simulink model "P4_F_sim"  (R2019a)
settings: Solver=VariableStepAuto  StartTime=0.0  StopTime=10.0  RelTol=1e-3
values from neighbouring files (symbols this model uses):
  A_AA = [ybb  yp+w0/u0 yr-1 g*ctt0/u0 ... (first row only)    [P3_F.m]
  B = [0    ydr ... (first row only)    [P3_F.m]
  bb_ref = 0.8    [P3_F.m]
  bb_stept = 10    [P3_F.m]
  C = eye(4)    [P3_F.m]
  D = zeros(4,2)    [P3_F.m]
  da0 = 0.58    [P3_F.m]
  damax = [-18 18]    [P3_F.m]
  deg = pi/180    (= 0.0174532925199)    [P3_F.m]
  dr0 = -0.01    [P3_F.m]
  drmax = [-23 23]    [P3_F.m]
  F = (CC*dcgain)^(-1)    [P3_F.m]
  K_lqr = lqr(A_AA,B,Q,R)    [P3_F.m]
  phi_ref = 15    [P3_F.m]
  phi_stept = 50    [P3_F.m]
libraries: simulink x4
settings Model: Creator=User  LastModifiedBy=User
settings DebuggingCC: SFMachineParentedDataDiag=error

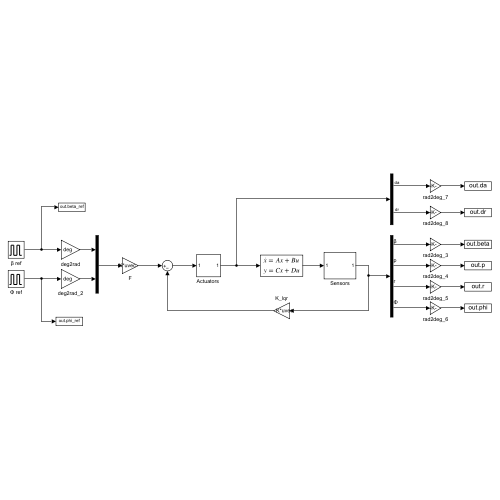
[thumbnail: Simulink's stored preview of the top-level diagram]
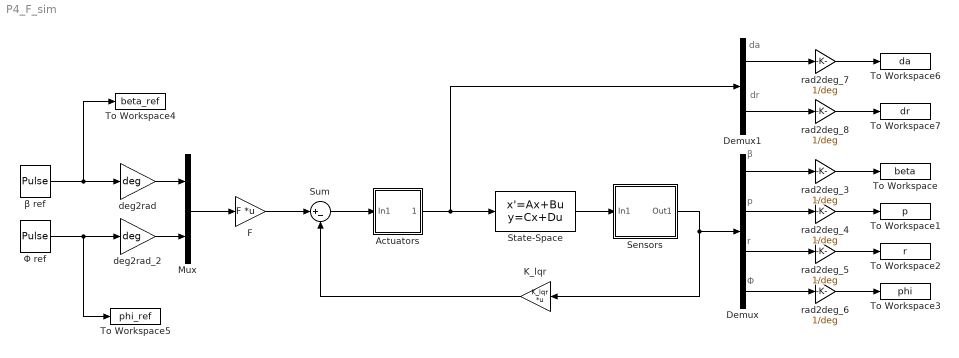
== system P4_F_sim ==
  note: r
  note: da
  note: p
  note: dr
  note: β
  note: Φ
  "Actuators " : Subsystem
  Demux : Demux
  Demux1 : Demux  Outputs=2
  F : Gain  Gain=F  Multiplication=Matrix(K*u) (u vector)
  K_lqr : Gain  Gain=K_lqr  Multiplication=Matrix(K*u) (u vector)
  Mux : Mux  Inputs=2
  Sensors : Subsystem
  State-Space : StateSpace  A=A_AA  B=B  C=C  D=D  InitialCondition=0
  Sum : Sum  Inputs=|+-
  To Workspace : ToWorkspace  VariableName=beta  SaveFormat=Timeseries  SampleTime=-1
  To Workspace1 : ToWorkspace  VariableName=p  SaveFormat=Timeseries  SampleTime=-1
  To Workspace2 : ToWorkspace  VariableName=r  SaveFormat=Timeseries  SampleTime=-1
  To Workspace3 : ToWorkspace  VariableName=phi  SaveFormat=Timeseries  SampleTime=-1
  To Workspace4 : ToWorkspace  VariableName=beta_ref  SaveFormat=Timeseries  SampleTime=-1
  To Workspace5 : ToWorkspace  VariableName=phi_ref  SaveFormat=Timeseries  SampleTime=-1
  To Workspace6 : ToWorkspace  VariableName=da  SaveFormat=Timeseries  SampleTime=-1
  To Workspace7 : ToWorkspace  VariableName=dr  SaveFormat=Timeseries  SampleTime=-1
  deg2rad : Gain  Gain=deg
  deg2rad_2 : Gain  Gain=deg
  rad2deg_{3..8} (6 alike) : Gain  Gain=1/deg
  Φ ref : DiscretePulseGenerator  PulseType=Time based  Amplitude=phi_ref  Period=100  PulseWidth=20  PhaseDelay=phi_stept
  β ref : DiscretePulseGenerator  PulseType=Time based  Amplitude=bb_ref  Period=100  PulseWidth=20  PhaseDelay=bb_stept
  wires:
  F/1 -> Sum/1
  Demux/2 -> rad2deg_4/1
  Demux/4 -> rad2deg_6/1
  Demux/3 -> rad2deg_5/1
  rad2deg_4/1 -> To Workspace1/1
  rad2deg_6/1 -> To Workspace3/1
  Demux1/1 -> rad2deg_7/1
  deg2rad/1 -> Mux/1
  rad2deg_7/1 -> To Workspace6/1
  K_lqr/1 -> Sum/2
  Mux/1 -> F/1
  Demux/1 -> rad2deg_3/1
  β ref/1 -> To Workspace4/1, deg2rad/1
  deg2rad_2/1 -> Mux/2
  rad2deg_8/1 -> To Workspace7/1
  Demux1/2 -> rad2deg_8/1
  rad2deg_5/1 -> To Workspace2/1
  rad2deg_3/1 -> To Workspace/1
  Φ ref/1 -> deg2rad_2/1, To Workspace5/1
  Sum/1 -> "Actuators "/1(In1)
  "Actuators "/1(Out1) -> Demux1/1, State-Space/1
  State-Space/1 -> Sensors/1(In1)
  Sensors/1(Out1) -> Demux/1, K_lqr/1

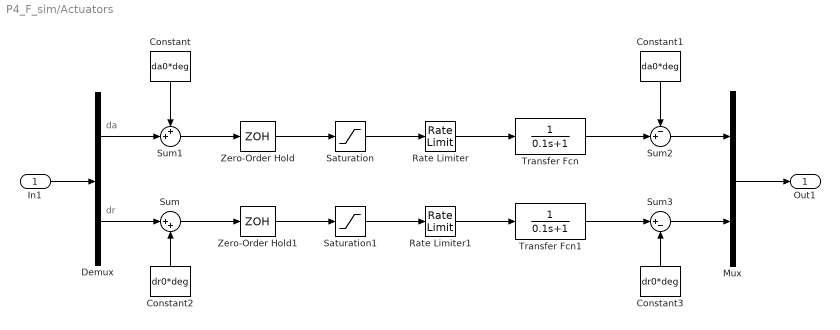
== system P4_F_sim/Actuators  ==
  note: da
  note: dr
  In1 : Inport
  Constant : Constant  Value=da0*deg
  Constant1 : Constant  Value=da0*deg
  Constant2 : Constant  Value=dr0*deg
  Constant3 : Constant  Value=dr0*deg
  Demux : Demux  Outputs=2
  Mux : Mux  Inputs=2
  Rate Limiter : RateLimiter  RisingSlewLimit=60*deg  FallingSlewLimit=-60*deg  SampleTimeMode=inherited
  Rate Limiter1 : RateLimiter  RisingSlewLimit=60*deg  FallingSlewLimit=-60*deg  SampleTimeMode=inherited
  Saturation : Saturate  UpperLimit=damax(2) * deg  LowerLimit=damax(1) * deg
  Saturation1 : Saturate  UpperLimit=drmax(2) * deg  LowerLimit=drmax(1) * deg
  Sum : Sum  Inputs=|++
  Sum1 : Sum  Inputs=++|
  Sum2 : Sum  Inputs=-+|
  Sum3 : Sum  Inputs=|+-
  Transfer Fcn : TransferFcn  Denominator=[0.1 1]
  Transfer Fcn1 : TransferFcn  Denominator=[0.1 1]
  Zero-Order Hold : ZeroOrderHold  SampleTime=0.025
  Zero-Order Hold1 : ZeroOrderHold  SampleTime=0.025
  Out1 : Outport
  wires:
  In1/1 -> Demux/1
  Zero-Order Hold/1 -> Saturation/1
  Zero-Order Hold1/1 -> Saturation1/1
  Saturation/1 -> Rate Limiter/1
  Saturation1/1 -> Rate Limiter1/1
  Rate Limiter/1 -> Transfer Fcn/1
  Rate Limiter1/1 -> Transfer Fcn1/1
  Mux/1 -> Out1/1
  Sum/1 -> Zero-Order Hold1/1
  Demux/2 -> Sum/1
  Sum1/1 -> Zero-Order Hold/1
  Demux/1 -> Sum1/2
  Transfer Fcn/1 -> Sum2/2
  Sum2/1 -> Mux/1
  Transfer Fcn1/1 -> Sum3/1
  Sum3/1 -> Mux/2
  Constant/1 -> Sum1/1
  Constant1/1 -> Sum2/1
  Constant3/1 -> Sum3/2
  Constant2/1 -> Sum/2

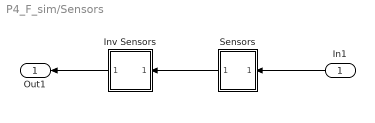
== system P4_F_sim/Sensors ==
  In1 : Inport
  Inv Sensors : Subsystem
  Sensors : Subsystem
  Out1 : Outport
  wires:
  Sensors/1(Out1) -> Inv Sensors/1(Input)
  Inv Sensors/1(Out1) -> Out1/1
  In1/1 -> Sensors/1(In1)

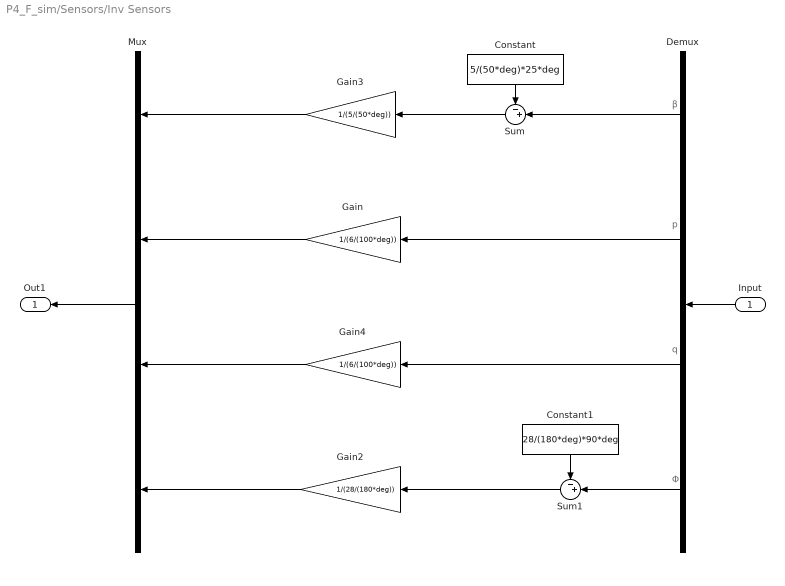
== system P4_F_sim/Sensors/Inv Sensors ==
  note: p
  note: β
  note: Φ
  note: q
  Input : Inport
  Constant : Constant  Value=5/(50*deg)*25*deg
  Constant1 : Constant  Value=28/(180*deg)*90*deg
  Demux : Demux
  Gain : Gain  Gain=1/(6/(100*deg))
  Gain2 : Gain  Gain=1/(28/(180*deg))
  Gain3 : Gain  Gain=1/(5/(50*deg))
  Gain4 : Gain  Gain=1/(6/(100*deg))
  Mux : Mux
  Sum : Sum  Inputs=-+|
  Sum1 : Sum  Inputs=-+|
  Out1 : Outport
  wires:
  Demux/4 -> Sum1/2
  Demux/2 -> Gain/1
  Mux/1 -> Out1/1
  Input/1 -> Demux/1
  Sum1/1 -> Gain2/1
  Gain3/1 -> Mux/1
  Constant/1 -> Sum/1
  Demux/1 -> Sum/2
  Sum/1 -> Gain3/1
  Demux/3 -> Gain4/1
  Constant1/1 -> Sum1/1
  Gain2/1 -> Mux/4
  Gain4/1 -> Mux/3
  Gain/1 -> Mux/2

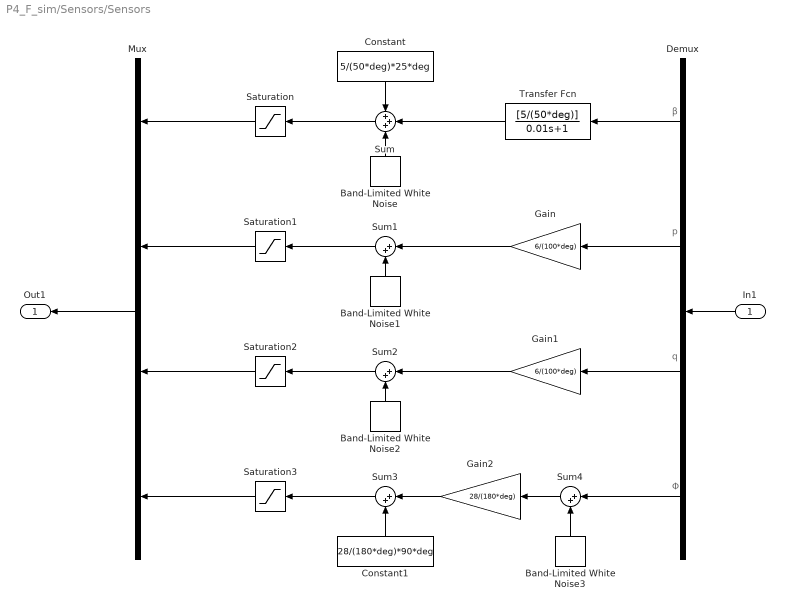
== system P4_F_sim/Sensors/Sensors ==
  note: β
  note: p
  note: q
  note: Φ
  In1 : Inport
  Band-Limited White Noise : simulink/Sources/Band-Limited White Noise  Cov=[0.005^2/40]  Ts=0.025  seed=[23341]
  Band-Limited White Noise1 : simulink/Sources/Band-Limited White Noise  Cov=[0.002^2/40]  Ts=0.025  seed=[23341]
  Band-Limited White Noise2 : simulink/Sources/Band-Limited White Noise  Cov=[0.002^2/40]  Ts=0.025  seed=[23341]
  Band-Limited White Noise3 : simulink/Sources/Band-Limited White Noise  Cov=[(0.25*deg)^2/40]  Ts=0.025  seed=[23341]
  Constant : Constant  Value=5/(50*deg)*25*deg
  Constant1 : Constant  Value=28/(180*deg)*90*deg
  Demux : Demux
  Gain : Gain  Gain=6/(100*deg)
  Gain1 : Gain  Gain=6/(100*deg)
  Gain2 : Gain  Gain=28/(180*deg)
  Mux : Mux
  Saturation : Saturate  UpperLimit=5  LowerLimit=0
  Saturation1 : Saturate  UpperLimit=3  LowerLimit=-3
  Saturation2 : Saturate  UpperLimit=3  LowerLimit=-3
  Saturation3 : Saturate  UpperLimit=28  LowerLimit=0
  Sum : Sum  Inputs=+++
  Sum{1..4} (4 alike) : Sum  Inputs=|++
  Transfer Fcn : TransferFcn  Numerator=[5/(50*deg)]  Denominator=[0.01 1]
  Out1 : Outport
  wires:
  In1/1 -> Demux/1
  Demux/1 -> Transfer Fcn/1
  Transfer Fcn/1 -> Sum/2
  Constant/1 -> Sum/1
  Band-Limited White Noise/1 -> Sum/3
  Sum/1 -> Saturation/1
  Saturation/1 -> Mux/1
  Mux/1 -> Out1/1
  Demux/2 -> Gain/1
  Gain/1 -> Sum1/1
  Band-Limited White Noise1/1 -> Sum1/2
  Sum1/1 -> Saturation1/1
  Saturation1/1 -> Mux/2
  Demux/3 -> Gain1/1
  Sum2/1 -> Saturation2/1
  Band-Limited White Noise2/1 -> Sum2/2
  Gain1/1 -> Sum2/1
  Saturation2/1 -> Mux/3
  Sum3/1 -> Saturation3/1
  Constant1/1 -> Sum3/2
  Gain2/1 -> Sum3/1
  Sum4/1 -> Gain2/1
  Demux/4 -> Sum4/1
  Saturation3/1 -> Mux/4
  Band-Limited White Noise3/1 -> Sum4/2
